simulink model "BBCCMonV1RLST1"  (Simulink 7.6)
settings: Solver=FixedStepDiscrete  StartTime=0.0  StopTime=5  FixedStep=1e-6  RelTol=1e-3
undefined symbols (not defined in the file): Imax, R, Ts, Vin
libraries: powerlib x12, powerlib_extras x2
settings Model: Creator=zxn  LastModifiedBy=zxn

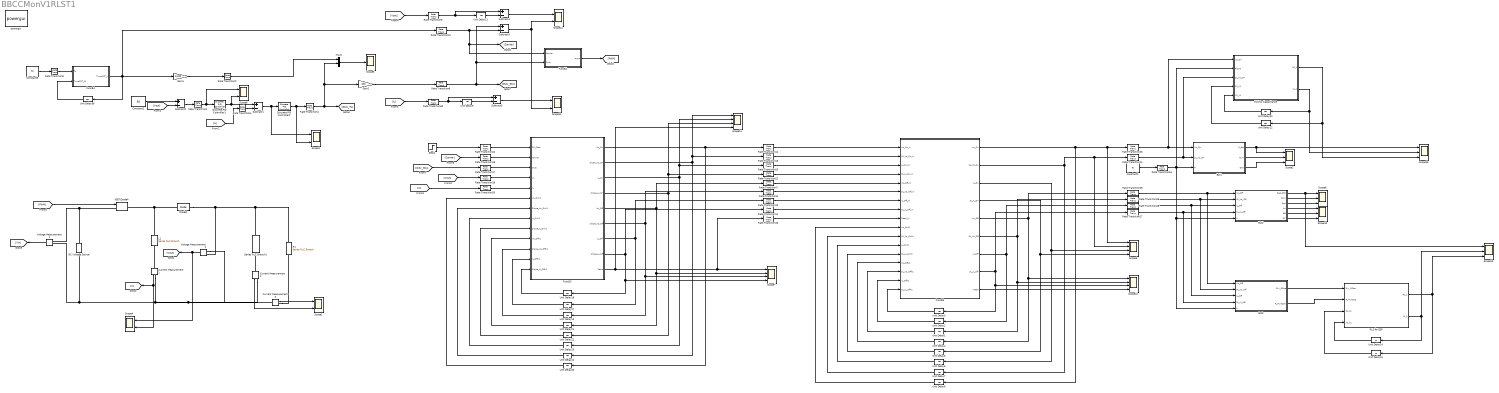
== system BBCCMonV1RLST1 ==
  Constant1 : Constant  Value=R
  Constant2 : Constant  Value=50
  Constant6 : Constant  Value=Ts
  Current Measurement1 : powerlib/Measurements/Current Measurement  DialogController=POWERSYS.PowerSysDialog  SystemSampleTime=-1  PhasorSimulation=off  OutputType=Complex  PSBequivalent=0
  Current Measurement2 : powerlib/Measurements/Current Measurement  DialogController=POWERSYS.PowerSysDialog  SystemSampleTime=-1  PhasorSimulation=off  OutputType=Complex  PSBequivalent=0
  Current Measurement3 : powerlib/Measurements/Current Measurement  DialogController=POWERSYS.PowerSysDialog  SystemSampleTime=-1  PhasorSimulation=off  OutputType=Complex  PSBequivalent=0
  DC Voltage Source : powerlib/Electrical Sources/DC Voltage Source  DialogController=POWERSYS.PowerSysDialog  SystemSampleTime=-1  Amplitude=Vin  Measurements=None
  Diode2 : powerlib/Power Electronics/Diode  DialogController=POWERSYS.PowerSysDialog  SystemSampleTime=-1  Ron=0.001  Lon=0  Vf=0.8  IC=0  UseSnubber=off  Rs=inf  Cs=inf  Measurements=off
  Discrete PID Controller1 : powerlib_extras/Discrete  Control Blocks/Discrete PID Controller  DialogController=POWERSYS.PowerSysDialog  SystemSampleTime=-1  Kp=1.4  Ki=0.4  Kd=0  TcD=0  Par_Limits=[1 -1]*Imax  Init=0  Ts=Ts
  Discrete PID Controller2 : powerlib_extras/Discrete  Control Blocks/Discrete PID Controller  DialogController=POWERSYS.PowerSysDialog  SystemSampleTime=-1  Kp=30e-3  Ki=50e-3  Kd=0  TcD=0  Par_Limits=[1 -1]*0.9  Init=0  Ts=Ts
  Est1 : Stateflow chart  TreatAsAtomicUnit=on
  Est2 : Stateflow chart  TreatAsAtomicUnit=on
  Est3 : Stateflow chart  TreatAsAtomicUnit=on
  FuncB1 : Stateflow chart  TreatAsAtomicUnit=on
  FuncB3 : Stateflow chart  TreatAsAtomicUnit=on
  FuncB4 : Stateflow chart  TreatAsAtomicUnit=on
  FuncB5 : Stateflow chart  TreatAsAtomicUnit=on
  Gain1 : Gain  Gain=1/100
  Gain2 : Gain  Gain=100
  IGBT/Diode4 : powerlib/Power Electronics/IGBT//Diode  DialogController=POWERSYS.PowerSysDialog  SystemSampleTime=-1  Ron=1e-3  Rs=1e5  Cs=inf  Measurements=off
  L1 : powerlib/Elements/Series RLC Branch  DialogController=POWERSYS.PowerSysDialog  PhysicalDomain=powersysdomain  SubClassName=unknown  LeftPortType=p1  RightPortType=p1  LConnTagsString=__new0  RConnTagsString=__new0  BranchType=L  Resistance=1  Inductance=5e-3  SetiL0=off  InitialCurrent=0  Capacitance=1e-6  Setx0=off  InitialVoltage=0  Measurements=None
  Mux5 : Mux  Inputs=2
  R1 : powerlib/Elements/Series RLC Branch  DialogController=POWERSYS.PowerSysDialog  PhysicalDomain=powersysdomain  SubClassName=unknown  LeftPortType=p1  RightPortType=p1  LConnTagsString=__new0  RConnTagsString=__new0  BranchType=R  Resistance=R  Inductance=1e-3  SetiL0=off  InitialCurrent=0  Capacitance=1e-6  Setx0=off  InitialVoltage=0  Measurements=None
  RLS for Capacitance : Stateflow chart  TreatAsAtomicUnit=on
  RLS for ESR : Stateflow chart  TreatAsAtomicUnit=on
  Rate Transition{1..2,6,8,12,15,17..21,30} (12 alike) : RateTransition  OutPortSampleTime=1e-6
  Rate Transition10 : RateTransition  X0=2.8  OutPortSampleTime=1e-6
  Rate Transition11 : RateTransition  X0=-1.2  OutPortSampleTime=1e-6
  Rate Transition13 : RateTransition  X0=-1  OutPortSampleTime=1e-6
  Rate Transition14 : RateTransition  X0=50  OutPortSampleTime=1e-6
  Rate Transition16 : RateTransition  X0=R  OutPortSampleTime=1e-6
  Rate Transition22 : RateTransition  X0=1.2  OutPortSampleTime=1e-6
  Rate Transition23 : RateTransition  X0=3  OutPortSampleTime=1e-6
  Rate Transition24 : RateTransition  X0=-1.2  OutPortSampleTime=1e-6
  Rate Transition25 : RateTransition  X0=50  OutPortSampleTime=1e-6
  Rate Transition26 : RateTransition  X0=1.2  OutPortSampleTime=1e-6
  Rate Transition27 : RateTransition  X0=-1  OutPortSampleTime=1e-6
  Rate Transition28 : RateTransition  X0=2.9  OutPortSampleTime=1e-6
  Rate Transition29 : RateTransition  X0=50.2  OutPortSampleTime=1e-6
  Rate Transition3 : RateTransition  OutPortSampleTime=Ts
  Rate Transition4 : RateTransition  OutPortSampleTime=Ts
  Rate Transition5 : RateTransition  X0=Ts  OutPortSampleTime=1e-6
  Rate Transition7 : RateTransition  X0=50.2  OutPortSampleTime=1e-6
  Rate Transition9 : RateTransition  X0=1  OutPortSampleTime=1e-6
  Scope{1,3..4,6,11..12} (6 alike) : Scope  NumInputPorts=2
      Scope1 settings: TickLabels=on  TimeRange=10  YMin=210~0  YMax=320~47.5  SaveName=var1
      Scope11 settings: TickLabels=on  TimeRange=5  YMin=-0.06~-40  YMax=0.07~65  SaveName=var10  MaxDataPoints=1000000
      Scope12 settings: TickLabels=on  TimeRange=5  YMin=-0.011~-40  YMax=0.01~65  SaveName=var13  MaxDataPoints=1000000
      Scope3 settings: TickLabels=on  TimeRange=1.5  YMin=0.5~0  YMax=0.605~1  SaveName=var4
      Scope4 settings: TickLabels=on  YMin=41.5~2.4  YMax=50~4.3  SaveName=var
      Scope6 settings: TickLabels=on  TimeRange=1.5  YMin=0.5~0  YMax=0.605~1  SaveName=var2
  Scope{7,9..10,14} (4 alike) : Scope  NumInputPorts=4
      Scope10 settings: TickLabels=on  TimeRange=5  YMin=-1~1.97916~47.5~0  YMax=1~2.1875~52.5~2  SaveName=var12  MaxDataPoints=1500000
      Scope14 settings: TickLabels=on  TimeRange=5  YMin=-1~1.97916~47.5~-1  YMax=1~2.1875~52.5~2  SaveName=var8  MaxDataPoints=1500000
      Scope7 settings: TickLabels=on  TimeRange=5  YMin=-1~1.97916~47.5~0  YMax=1~2.1875~52.5~2  SaveName=var11  MaxDataPoints=1500000
      Scope9 settings: TickLabels=on  TimeRange=5  YMin=-1~1.97916~47.5~0  YMax=1~2.1875~52.5~2  SaveName=var9  MaxDataPoints=1500000
  Scope{2,8,13,15..16} (5 alike) : Scope  NumInputPorts=3
      Scope13 settings: TickLabels=on  TimeRange=5  YMin=3.675~49.875~0.0079992  YMax=4.025~50.125~0.00799926  SaveName=var3  MaxDataPoints=1000000
      Scope15 settings: TickLabels=on  TimeRange=5  YMin=0~0~0.0079992  YMax=0.1~0.1~0.00799926  SaveName=var14  MaxDataPoints=1000000
      Scope16 settings: TickLabels=on  TimeRange=3  YMin=8.3e-005~0.66~7998.55  YMax=9.05e-005~0.725~7998.68  SaveName=var15  MaxDataPoints=1000000
      Scope2 settings: TickLabels=on  TimeRange=3  YMin=8.3e-005~0.66~7998.55  YMax=9.05e-005~0.725~7998.68  SaveName=var6  MaxDataPoints=1000000
      Scope8 settings: TickLabels=on  TimeRange=5  YMin=3.675~49.875~0.0079992  YMax=4.025~50.125~0.00799926  SaveName=var7  MaxDataPoints=1000000
  Scope5 : Scope
      settings: TickLabels=on  TimeRange=1.5  YMin=0.5  YMax=0.605  SaveName=var5  MaxDataPoints=100000
  Series RLC Branch1 : powerlib/Elements/Series RLC Branch  DialogController=POWERSYS.PowerSysDialog  PhysicalDomain=powersysdomain  SubClassName=unknown  LeftPortType=p1  RightPortType=p1  LConnTagsString=__new0  RConnTagsString=__new0  BranchType=RC  Resistance=75e-3*1  Inductance=1e-3  SetiL0=off  InitialCurrent=0  Capacitance=1e-3*1.25  Setx0=off  InitialVoltage=500  Measurements=None
  Step1 : Step  Time=3.3  SampleTime=0
  Subtract1 : Sum  Inputs=+-  SampleTime=Ts
  Subtract{2..5} (4 alike) : Sum  Inputs=+-
  Unit Delay{1..15,17..18,21..25,56} (23 alike) : UnitDelay  SampleTime=1e-6
  Voltage Measurement1 : powerlib/Measurements/Voltage Measurement  DialogController=POWERSYS.PowerSysDialog  SystemSampleTime=-1  PhasorSimulation=off  OutputType=Complex  PSBequivalent=0
  Voltage Measurement2 : powerlib/Measurements/Voltage Measurement  DialogController=POWERSYS.PowerSysDialog  SystemSampleTime=-1  PhasorSimulation=off  OutputType=Complex  PSBequivalent=0
  powergui : powerlib/powergui  Priority=2  SystemSampleTime=-1  SimulationMode=Discrete  SampleTime=1e-6  frequency=60  SPID=off  DisableSnubberDevices=off  DisableRonSwitches=off  DisableVfSwitches=off  SwTol=0  Interpol=off  frequencyindice=0  echomessages=off  HookPort=off  DisplayEquations=off  FunctionMessages=off  EnableUseOfTLC=off  x0status=blocks  RestoreLinks=warning  ResistiveCurrentMeasurement=off  Frange=[0:2:500]  Ylog=off  Xlog=off  ShowGrid=off  save=off  variable=ZData  structure=ScopeData  ZoomFFT=on  StartTime=0.0  cycles=1  DisplayStyle=1  fundamental=60  FreqAxis=off  MaxFrequency=8000  frequencyindicesteady=1  RmsSteady=1  display=off  Ts=0  methode=off
  wires:
  Constant2/1 -> Subtract2/1
  Subtract2/1 -> Rate Transition3/1
  Voltage Measurement2/1 -> Scope4/1, [Vout]
  Current Measurement1/1 -> [IL], Scope4/2
  Current Measurement3/1 -> Scope1/1
  Current Measurement2/1 -> Scope1/2
  Rate Transition2/1 -> Mux5/1
  Rate Transition3/1 -> Discrete PID Controller1/1, Scope6/1
  Discrete PID Controller1/1 -> Subtract1/1, Scope6/2
  Subtract1/1 -> Discrete PID Controller2/1, Scope3/1
  Rate Transition4/1 -> Subtract1/2
  [IL] -> Rate Transition4/1
  [Vout] -> Subtract2/2
  Discrete PID Controller2/1 -> Rate Transition1/1, Scope3/2
  Rate Transition1/1 -> Mux5/2, Gain2/1, [Duty_Ts]
  Mux5/1 -> Scope5/1
  Rate Transition6/1 -> [Duty_SCL], Subtract3/1, FuncB1/2(Duty)
  Rate Transition8/1 -> Unit Delay11/1, Subtract4/1
  [PWM] -> IGBT/Diode4/1
  Voltage Measurement1/1 -> [Vin]
  Rate Transition5/1 -> FuncB4/1(Ts)
  Constant6/1 -> Rate Transition5/1
  Unit Delay56/1 -> FuncB4/2(TimeCNT_k1)
  FuncB4/1(TimeCNT_k) -> Unit Delay56/1, Gain1/1, Rate Transition12/1
  Gain1/1 -> Rate Transition2/1
  Gain2/1 -> Rate Transition6/1
  Subtract3/1 -> Scope11/2, Scope12/2
  Rate Transition12/1 -> Subtract3/2, [Carrier], FuncB1/1(Carrier)
  Unit Delay11/1 -> Subtract4/2
  Subtract4/1 -> Scope11/1
  [Vout] -> Rate Transition8/1
  [Carrier] -> Rate Transition18/1
  [Duty_SCL] -> Rate Transition17/1
  Step1/1 -> Rate Transition21/1
  [IL] -> Rate Transition20/1
  [Vout] -> Rate Transition19/1
  FuncB1/1(PWM) -> [PWM]
  Rate Transition21/1 -> FuncB3/1(SS_Start)
  Rate Transition18/1 -> FuncB3/2(Carrier)
  Rate Transition17/1 -> FuncB3/3(Duty)
  Rate Transition19/1 -> FuncB3/4(Vc)
  Rate Transition20/1 -> FuncB3/5(IL)
  FuncB3/8(Slope_IL_Off) -> Rate Transition11/1, Unit Delay18/1, Scope7/4
  Unit Delay18/1 -> FuncB3/13(Slope_IL_Offk1)
  FuncB3/7(IL_Off) -> Unit Delay17/1, Rate Transition10/1
  FuncB3/6(Slope_Vo_Off) -> Rate Transition9/1, Unit Delay13/1, Scope7/3
  Unit Delay17/1 -> FuncB3/12(IL_Offk1)
  Unit Delay13/1 -> FuncB3/11(Slope_Vo_Offk1)
  FuncB3/5(Vo_Off) -> Rate Transition7/1, Unit Delay21/1, Scope7/2
  Unit Delay21/1 -> FuncB3/10(Vo_Offk1)
  FuncB3/4(Slope_IL_On) -> Unit Delay22/1, Rate Transition22/1, Scope14/3
  Unit Delay22/1 -> FuncB3/9(Slope_IL_Onk1)
  FuncB3/3(IL_On) -> Unit Delay23/1, Rate Transition23/1, Scope14/2
  Unit Delay23/1 -> FuncB3/8(IL_Onk1)
  FuncB3/2(Slope_Vo_On) -> Unit Delay24/1, Rate Transition13/1, Scope14/1
  FuncB3/1(Vo_On) -> Unit Delay25/1, Rate Transition14/1
  Unit Delay24/1 -> FuncB3/7(Slope_Vo_Onk1)
  Unit Delay25/1 -> FuncB3/6(Vo_Onk1)
  Rate Transition14/1 -> FuncB5/1(Vo_On_In)
  Rate Transition13/1 -> FuncB5/2(SL_Vo_On_In)
  Rate Transition23/1 -> FuncB5/3(IL_On_In)
  Rate Transition22/1 -> FuncB5/4(SL_IL_On_In)
  Rate Transition7/1 -> FuncB5/5(Vo_Off_In)
  Rate Transition9/1 -> FuncB5/6(SL_Vo_Off_In)
  Rate Transition10/1 -> FuncB5/7(IL_Off_In)
  Rate Transition11/1 -> FuncB5/8(SL_IL_Off_In)
  Est1/2(Num) -> Scope2/2
  Est1/1(C_Est) -> Scope2/1, Scope16/1
  Est1/3(Den) -> Scope2/3
  Est2/3(Den) -> Scope8/3
  Est2/2(Num) -> Scope8/2
  Est2/1(Resr_Est) -> Scope8/1, Scope15/1
  Est2/4(AA) -> Scope13/1
  FuncB5/8(SL_IL_Off) -> Rate Transition27/1, Unit Delay3/1, Scope10/3
  FuncB5/7(IL_Off) -> Unit Delay2/1, Rate Transition28/1
  Unit Delay3/1 -> FuncB5/17(SL_IL_Offk1)
  Unit Delay2/1 -> FuncB5/16(IL_Offk1)
  FuncB5/6(SL_Vo_Off) -> Rate Transition26/1, Unit Delay1/1, Scope10/2
  Unit Delay1/1 -> FuncB5/15(SL_Vo_Offk1)
  FuncB5/5(Vo_Off) -> Rate Transition29/1, Unit Delay4/1, Scope10/1
  Unit Delay4/1 -> FuncB5/14(Vo_Offk1)
  FuncB5/4(SL_IL_On) -> Unit Delay5/1, Scope9/4
  Unit Delay5/1 -> FuncB5/13(SL_IL_Onk1)
  FuncB5/3(IL_On) -> Unit Delay6/1, Scope9/3
  FuncB5/2(SL_Vo_On) -> Unit Delay7/1, Rate Transition24/1, Scope9/2
  Unit Delay6/1 -> FuncB5/12(IL_Onk1)
  Unit Delay7/1 -> FuncB5/11(SL_Vo_Onk1)
  FuncB5/1(Vo_On) -> Unit Delay8/1, Rate Transition25/1, Scope9/1
  Unit Delay8/1 -> FuncB5/10(Vo_Onk1)
  Rate Transition15/1 -> FuncB5/9(Read_In)
  FuncB3/9(Read) -> Rate Transition15/1, Scope7/1, Scope14/4
  Constant1/1 -> Rate Transition16/1
  Rate Transition25/1 -> Est1/1(Vo_On), RLS for Capacitance/1(Vo_On)
  Rate Transition24/1 -> Est1/2(SL_Vo_On), RLS for Capacitance/3(SL_Vo_On)
  Rate Transition16/1 -> Est1/3(R), Est2/5(R), Est3/5(R), RLS for Capacitance/2(Rload)
  Est2/5(BB) -> Scope13/2
  Est2/6(CC) -> Scope13/3
  Rate Transition26/1 -> Est2/2(SL_Vo_Off), Est3/2(SL_Vo_Off)
  Rate Transition27/1 -> Est2/4(SL_IL_Off), Est3/4(SL_IL_Off)
  Rate Transition28/1 -> Est2/3(IL_Off), Est3/3(IL_Off)
  Rate Transition29/1 -> Est2/1(Vo_Off), Est3/1(Vo_Off)
  FuncB5/9(Read) -> Scope10/4
  [IL] -> Rate Transition30/1
  Unit Delay9/1 -> Subtract5/2
  Rate Transition30/1 -> Unit Delay9/1, Subtract5/1
  Subtract5/1 -> Scope12/1
  Est3/1(Div_RCoe) -> RLS for ESR/1(Div_RCoe)
  Est3/2(R_MultCoe) -> RLS for ESR/2(R_MultCoe)
  RLS for Capacitance/2(X1_k) -> Unit Delay10/1, Scope16/2
  Unit Delay10/1 -> RLS for Capacitance/5(X1_k1)
  RLS for Capacitance/1(R1_k) -> Unit Delay12/1, Scope16/3
  Unit Delay12/1 -> RLS for Capacitance/4(R1_k1)
  RLS for ESR/2(X1_k) -> Unit Delay14/1, Scope15/2
  Unit Delay14/1 -> RLS for ESR/4(X1_k1)
  RLS for ESR/1(R1_k) -> Unit Delay15/1, Scope15/3
  Unit Delay15/1 -> RLS for ESR/3(R1_k1)
  connections:
  DC Voltage Source/RConn1 -- IGBT/Diode4/LConn1 -- Voltage Measurement1/LConn1
  Diode2/RConn1 -- IGBT/Diode4/RConn1 -- L1/RConn1
  Current Measurement3/LConn1 -- Current Measurement2/RConn1 -- Voltage Measurement2/LConn1 -- Current Measurement1/RConn1 -- DC Voltage Source/LConn1 -- Voltage Measurement1/LConn2
  Current Measurement1/LConn1 -- L1/LConn1
  Diode2/LConn1 -- R1/RConn1 -- Series RLC Branch1/RConn1 -- Voltage Measurement2/LConn2
  Current Measurement2/LConn1 -- Series RLC Branch1/LConn1
  Current Measurement3/RConn1 -- R1/LConn1

== matlab function Est1 ==
  data: Vo_On input double; SL_Vo_On input double; R input double; C_Est output double; Num output double; Den output double
function [C_Est,Num,Den] = OnState(Vo_On,SL_Vo_On,R)

Num=-Vo_On/R; %%*0.5
Den=SL_Vo_On;
C_Temp=Num/Den;
%if(Resr_Temp>=Resr_Est_k1)
%    Resr_Est=Resr_Est_k1;
%else
    C_Est=C_Temp;
%end

end

== matlab function FuncB3 ==
  data: SS_Start input double; Carrier input double; Duty input double; Vc input double; IL input double; Vo_Onk1 input double; Slope_Vo_Onk1 input double; IL_Onk1 input double; Slope_IL_Onk1 input double; Vo_Offk1 input double; Slope_Vo_Offk1 input double; IL_Offk1 input double; Vo_On output double; Slope_Vo_On output double; IL_On output double; Slope_IL_On output double; Vo_Off output double; Slope_Vo_Off output double; IL_Off output double; Slope_IL_Off output double; Read output double; Slope_IL_Offk1 input double
function [Vo_On,Slope_Vo_On,IL_On,Slope_IL_On,Vo_Off,Slope_Vo_Off,IL_Off,Slope_IL_Off,Read] = Sample(SS_Start,Carrier,Duty,Vc,IL,Vo_Onk1,Slope_Vo_Onk1,IL_Onk1,Slope_IL_Onk1,Vo_Offk1,Slope_Vo_Offk1,IL_Offk1,Slope_IL_Offk1)

Err1=(Carrier - Duty);  Tsimulation=1e-6;
%DtT_On=Duty*Tsimulation;    DtT_Off=(100 - Duty)*Tsimulation;%%!! 100 should be repaced Correspondingly by CNT_Max
Fix10us=10e-6;
if(SS_Start==1)
    if(Err1>=-12)&&(Err1<-11) %%Just After Switch-On; (Err1>=-2)&&(Err1<-1); (Carrier==3)
        Vo_On=Vc; IL_On=IL;
        Read=0;
        Slope_Vo_On=Slope_Vo_Onk1; Slope_IL_On=Slope_IL_Onk1;
        Slope_Vo_Off=Slope_Vo_Offk1; Slope_IL_Off=Slope_IL_Offk1;
        Vo_Off=Vo_Offk1; IL_Off=IL_Offk1;
    elseif((Err1>=-2)&&(Err1<-1)) %%Next moment Switch-Off
        %Slope_Vo_On=(Vc - Vo_Onk1)/DtT_On; Slope_IL_On=(IL - IL_Onk1)/DtT_On;
        Slope_Vo_On=(Vc - Vo_Onk1)/Fix10us; Slope_IL_On=(IL - IL_Onk1)/Fix10us;
        Vo_On=Vo_Onk1; IL_On=IL_Onk1;
        Slope_Vo_Off=Slope_Vo_Offk1; Slope_IL_Off=Slope_IL_Offk1; Read=0; 
        Vo_Off=Vo_Offk1; IL_Off=IL_Offk1;
    elseif(Carrier==89) %%Just After Switch Off; Carrier==98; (Err1>3)&&(Err1<=4)
        Vo_Off=Vc;  IL_Off=IL;
        Slope_Vo_Off=Slope_Vo_Offk1;  Slope_IL_Off=Slope_IL_Offk1;
        Slope_Vo_On=Slope_Vo_Onk1;  Slope_IL_On=Slope_IL_Onk1; Read=0;
        Vo_On=Vo_Onk1; IL_On=IL_Onk1;
    elseif(Carrier==99) %%Next moment Switch-On
        %Slope_Vo_Off=(Vc - Vo_Offk1)/DtT_Off;  Slope_IL_Off=(IL - IL_Offk1)/DtT_Off;
        Slope_Vo_Off=(Vc - Vo_Offk1)/Fix10us;  Slope_IL_Off=(IL - IL_Offk1)/Fix10us;
        Vo_Off=Vo_Offk1;  IL_Off=IL_Offk1;
        Read=1;
        Slope_Vo_On=Slope_Vo_Onk1; Slope_IL_On=Slope_IL_Onk1;
        Vo_On=Vo_Onk1; IL_On=IL_Onk1;
    else
        Vo_On=Vo_Onk1; Slope_Vo_On=Slope_Vo_Onk1; IL_On=IL_Onk1; Slope_IL_On=Slope_IL_Onk1; %%On_Readk1
        Vo_Off=Vo_Offk1;  Slope_Vo_Off=Slope_Vo_Offk1;  IL_Off=IL_Offk1;  Slope_IL_Off=Slope_IL_Offk1; Read=0; %%Off_Readk1
    end
else
    Vo_On=49;  Slope_Vo_On=0.5;  IL_On=4;  Slope_IL_On=0.2;
    Vo_Off=50;  Slope_Vo_Off=0.5;  IL_Off=3.8;  Slope_IL_Off=0.2; Read=0;
end

end

== matlab function RLS for Capacitance ==
  data: Vo_On input double; Rload input double; SL_Vo_On input double; R1_k output double; R1_k1 input double; X1_k output double; X1_k1 input double
function [R1_k,X1_k] = FRLS1(Vo_On,Rload,SL_Vo_On,R1_k1,X1_k1)
%%Algorithm Initialization
%%X=lspr(Dt_ISlope,Dt_Vap,0.95)--Better
Lamda=0.9982; %%0.9999
Ic_In=-Vo_On/Rload;
Vo_Slope=SL_Vo_On;
Err_k=Ic_In - Vo_Slope*X1_k1;
%%[R,yb]=newqr(R1_k1,X1_k1,phi,Err_k,Lamda);
[m1,n1]=size(R1_k1);
BigR=[R1_k1,0;
      Vo_Slope,Err_k];
for i=1:n1
   %%[m2,n2]=size(BigR);
   n2=2;
   %%[c,s,r]=givens(BigR(i,i)*lam,BigR(n2,i));
   a=BigR(i,i)*Lamda;  b=BigR(n2,i);
   r=sqrt(a^2 + b^2);
   if(r<1e-8)%%r<1e-8
     c=1; s=0; r=1e-8; %%r=1e-8
   else
     c=a/r; s=b/r; 
   end
   %%end of 'givens' => Continue of 'sweep'
   BigR(i,i)=r;
   BigR(n2,i)=0.0;
   clam=c*Lamda;
   slam=s*Lamda;
   for k=i+1:n2
      a=BigR(i,k)*clam + BigR(n2,k)*s;
      BigR(n2,k)=-BigR(i,k)*slam + BigR(n2,k)*c;
      BigR(i,k)=a;
   end
end
%%end of 'sweep'
R=BigR(1:n1,1:n1);
yb=BigR(1:n1,n1+1);
%%end of 'newqr'
dx=0.0;
%%dx=solve(X1_k1,R,yb);
%%??? Investigate RLS, here how to modify ??? Is it just by setting sum=0
%%at 'else' sentence
dx(1,1)=(yb)/R;
%%end of 'solve'
X_k=X1_k1 + dx;
%%Value Distribution After Computation
R1_k=R;
X1_k=X_k;

end

== matlab function FuncB5 ==
  data: Vo_On output double; Vo_On_In input double; SL_Vo_On_In input double; IL_On_In input double; SL_IL_On_In input double; Vo_Off_In input double; SL_Vo_Off_In input double; IL_Off_In input double; SL_IL_Off_In input double; Read_In input double; Vo_Onk1 input double; SL_Vo_Onk1 input double; IL_Onk1 input double; SL_IL_Onk1 input double; Vo_Offk1 input double; SL_Vo_On output double; IL_On output double; SL_IL_On output double; Vo_Off output double; SL_Vo_Off output double; IL_Off output double; SL_IL_Off output double; Read output double; SL_Vo_Offk1 input double; IL_Offk1 input double; SL_IL_Offk1 input double
function [Vo_On,SL_Vo_On,IL_On,SL_IL_On,Vo_Off,SL_Vo_Off,IL_Off,SL_IL_Off,Read] = Sample(Vo_On_In,SL_Vo_On_In,IL_On_In,SL_IL_On_In,Vo_Off_In,SL_Vo_Off_In,IL_Off_In,SL_IL_Off_In,Read_In,Vo_Onk1,SL_Vo_Onk1,IL_Onk1,SL_IL_Onk1,Vo_Offk1,SL_Vo_Offk1,IL_Offk1,SL_IL_Offk1)

if(Read_In==1)
    Vo_On=Vo_On_In; IL_On=IL_On_In;
    Vo_Off=Vo_Off_In;  SL_Vo_Off=SL_Vo_Off_In;  IL_Off=IL_Off_In;  SL_IL_Off=SL_IL_Off_In; Read=Read_In;
    if((SL_Vo_On_In>-1300)||(SL_Vo_On_In<-1350))
        SL_Vo_On=SL_Vo_Onk1;
    else
        SL_Vo_On=SL_Vo_On_In;
    end
    if((SL_IL_On_In>8500)||(SL_IL_On_In<7500))
        SL_IL_On=SL_IL_Onk1;
    else
        SL_IL_On=SL_IL_On_In;
    end
else
    Vo_On=Vo_Onk1;  SL_Vo_On=SL_Vo_Onk1;  IL_On=IL_Onk1;  SL_IL_On=SL_IL_Onk1;
    Vo_Off=Vo_Offk1;  SL_Vo_Off=SL_Vo_Offk1;  IL_Off=IL_Offk1;  SL_IL_Off=SL_IL_Offk1; Read=0;
end

end

== matlab function RLS for ESR ==
  data: Div_RCoe input double; R_MultCoe input double; R1_k output double; R1_k1 input double; X1_k output double; X1_k1 input double
function [R1_k,X1_k] = FRLS1(Div_RCoe,R_MultCoe,R1_k1,X1_k1)
%%Algorithm Initialization
%%X=lspr(Dt_ISlope,Dt_Vap,0.95)--Better
Lamda=0.9982; %%0.9999
Err_k=Div_RCoe - R_MultCoe*X1_k1;
%%[R,yb]=newqr(R1_k1,X1_k1,phi,Err_k,Lamda);
[m1,n1]=size(R1_k1);
BigR=[R1_k1,0;
      R_MultCoe,Err_k];
for i=1:n1
   %%[m2,n2]=size(BigR);
   n2=2;
   %%[c,s,r]=givens(BigR(i,i)*lam,BigR(n2,i));
   a=BigR(i,i)*Lamda;  b=BigR(n2,i);
   r=sqrt(a^2 + b^2);
   if(r<1e-8)%%r<1e-8
     c=1; s=0; r=1e-8; %%r=1e-8
   else
     c=a/r; s=b/r; 
   end
   %%end of 'givens' => Continue of 'sweep'
   BigR(i,i)=r;
   BigR(n2,i)=0.0;
   clam=c*Lamda;
   slam=s*Lamda;
   for k=i+1:n2
      a=BigR(i,k)*clam + BigR(n2,k)*s;
      BigR(n2,k)=-BigR(i,k)*slam + BigR(n2,k)*c;
      BigR(i,k)=a;
   end
end
%%end of 'sweep'
R=BigR(1:n1,1:n1);
yb=BigR(1:n1,n1+1);
%%end of 'newqr'
dx=0.0;
%%dx=solve(X1_k1,R,yb);
%%??? Investigate RLS, here how to modify ??? Is it just by setting sum=0
%%at 'else' sentence
dx(1,1)=(yb)/R;
%%end of 'solve'
X_k=X1_k1 + dx;
%%Value Distribution After Computation
R1_k=R;
X1_k=X_k;

end

== matlab function Est2 ==
  data: Vo_Off input double; SL_Vo_Off input double; IL_Off input double; SL_IL_Off input double; R input double; Resr_Est output double; Num output double; Den output double; AA output double; BB output double; CC output double
function [Resr_Est,Num,Den,AA,BB,CC] = OffState(Vo_Off,SL_Vo_Off,IL_Off,SL_IL_Off,R)

C=1e-3*1.25;
AA=C*SL_Vo_Off;  BB=-IL_Off;  CC=Vo_Off/R;
Num=AA + BB + CC; %%*0.5
DD=SL_IL_Off;  EE=-1/R*SL_Vo_Off;
Den=(DD + EE)*C;
Resr_Temp=Num/Den;
%if(Resr_Temp>=Resr_Est_k1)
%    Resr_Est=Resr_Est_k1;
%else
    Resr_Est=Resr_Temp;
%end

end

== matlab function Est3 ==
  data: Vo_Off input double; SL_Vo_Off input double; IL_Off input double; SL_IL_Off input double; R input double; Div_RCoe output double; R_MultCoe output double
function [Div_RCoe,R_MultCoe] = OffState(Vo_Off,SL_Vo_Off,IL_Off,SL_IL_Off,R)

C=1e-3*1.25;
AA=C*SL_Vo_Off;  BB=-IL_Off;  CC=Vo_Off/R;
Div_RCoe=AA + BB + CC; %%*0.5
DD=SL_IL_Off;  EE=-1/R*SL_Vo_Off;
R_MultCoe=(DD + EE)*C;

end

== matlab function FuncB1 ==
  data: PWM output double; Carrier input double; Duty input double
function PWM  = Sample(Carrier,Duty)

Err1=(Duty - Carrier);
%%Single Switch PWM Signal Generation!
if(Err1>0)
    PWM=1;
else
    PWM=0;
end

end

== matlab function FuncB4 ==
  data: Ts input double; TimeCNT_k1 input double; TimeCNT_k output double
function TimeCNT_k  = IabSlope(Ts,TimeCNT_k1)

Tsimulation=1e-6;
CNT_Ts=Ts/Tsimulation - 1; %%100
%%Vap,Vbt Calculation
if(TimeCNT_k1>=CNT_Ts)
    TimeCNT_k=0;
else
    TimeCNT_k=TimeCNT_k1 + 1;
end

end
